simulink library "others"  (R2014a)
settings: Solver=ode45  StartTime=0.0  StopTime=10.0  RelTol=1e-3
undefined symbols (not defined in the file): n, num_closest_obstacles, TadjacencyMatrix, Tsim
settings Model: Creator=rspica  LastModifiedBy=rspica

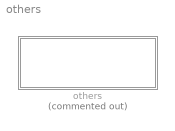
== system others ==
  others : Subsystem  Commented=on

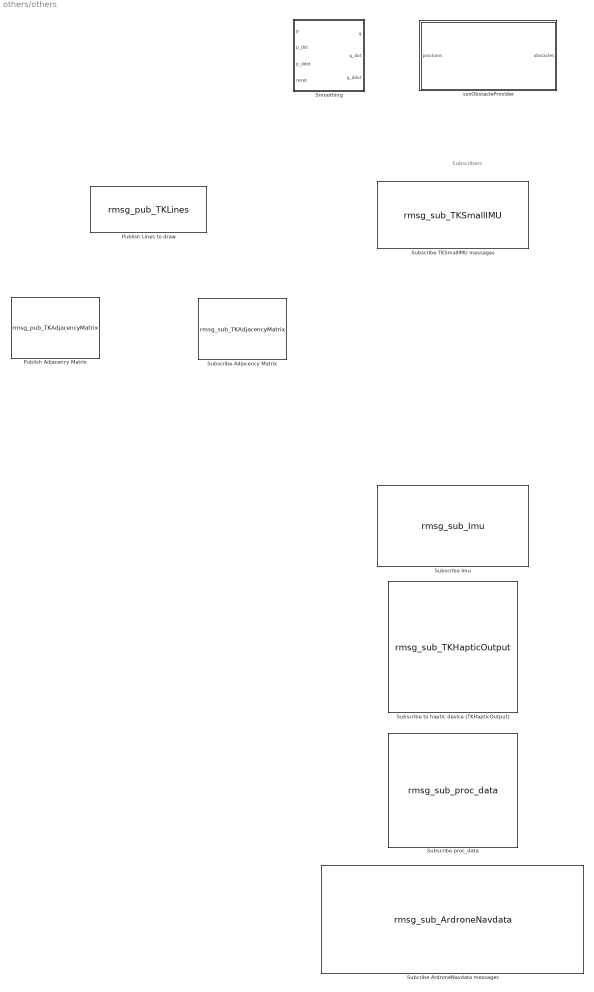
== system others/others ==
  note: Subscribers
  Publish Adjacency Matrix : S-Function  FunctionName=rmsg_pub_TKAdjacencyMatrix  Parameters=stepTime,topic  EnableBusSupport=off  mask{stepTime=TadjacencyMatrix, topic='/Matlab/AdjacencyMatrix'}
      mask prompts: stepTime "Simulation time step"; topic "ROS Topic"
      mask Display:
      | disp('Publish an\n\nAdjacency Matrix')
      | port_label('input', 1, 'A')
  Publish Lines to draw : S-Function  FunctionName=rmsg_pub_TKLines  Parameters=stepTime,topic  EnableBusSupport=off  mask(Line Drawer){stepTime=Tsim, topic='/TeleKyb/SwarmSimX/LineDrawer/input'}
      mask prompts: stepTime "Simulation time step"; topic "ROS Topic"
      mask help: This Block posts a collection of lines to the given ROS-Topic. Each line consists of a start- and destination-point in 3D and a color in 3D as RGB.
      mask Display:
      | disp('Line\nDrawer')
      | port_label('input', 1, 'start')
      | port_label('input', 2, 'destination')
      | port_label('input', 3, 'color')
  Smoothing : Subsystem  mask{time_to_95_percent=0.2}
      mask prompts: time_to_95_percent "Time in which 95% tracking should be reached"
      mask init:
      | A_smoothing = [0 0 0 0; 1 0 0 0; 0 1 0 0; 0 0 1 0];
      | B_smoothing = [1; 0; 0; 0];
      | dominant_pole = -3/time_to_95_percent;
      | p_smoothing = [dominant_pole, dominant_pole-1, dominant_pole-2, dominant_pole-3];
      | k_tracking = place(A_smoothing, B_smoothing, p_smoothing);
  "Subcribe ArdroneNavdata messages " : S-Function  FunctionName=rmsg_sub_ArdroneNavdata  Parameters=stepTime,topic_prefix,list_of_ids,topic_postfix  EnableBusSupport=off  mask{stepTime=Tsim, topic_prefix='/ardrone_', list_of_ids=uint32([0 1 2 3]), topic_postfix='/navdata'}
      mask prompts: stepTime "Simulation time step"; topic_prefix "ROS Topic (Prefix)"; list_of_ids "List of robot IDs (must be a vector of uint32)"; topic_postfix "ROS Topic (Postfix)"
      mask Display:
      | disp('Subscriber to \n ArdroneNavdata messages')
      | port_label('output',1,'magnetometer')
      | port_label('output',2,'pressure')
      | port_label('output',3,'temperature')
      | port_label('output',4,'rotation [degree angles]')
      | port_label('output',5,'altitude [cm]')
      | port_label('output',6,'velocity [mm/s]')
      | port_label('output',7,'raw vision velocity [mm/s]')
      | port_label('output',8,'accelerometers [g]')
      | port_label('output',9,'gyroscopes [deg/s]')
      | port_label('output',10,'vision state')
      | port_label('output',11,'state')
      | port_label('output',12,'battery level [%]')
      | port_label('output',13,'wind info')
      | port_label('output',14,'internal time')
      | port_label('output',15,'sent time')
  Subscribe Adjacency Matrix : S-Function  FunctionName=rmsg_sub_TKAdjacencyMatrix  Parameters=stepTime,topic,numRobots  EnableBusSupport=off  mask{stepTime=TadjacencyMatrix, topic='/Matlab/AdjacencyMatrix', numRobots=n}
      mask prompts: stepTime "Simulation time step"; topic "ROS Topic"; numRobots "number of robots"
      mask Display:
      | disp('Subscribe to\nAdjacency Matrix')
      | port_label('output', 1, 'A')
      | port_label('output', 2, 'sent time')
  Subscribe Imu : S-Function  FunctionName=rmsg_sub_Imu  Parameters=stepTime, topic_prefix,list_of_robot_ids,topic_postfix  EnableBusSupport=off  mask(Subscriber TKState){stepTime=Tsim, topic_prefix='/TeleKyb/SwarmSimX/Mikrokopter', list_of_robot_ids=uint32([0 1 2 3]), topic_postfix='/Sensor/VirtualIMU'}
      mask prompts: stepTime "Simulation time step"; topic_prefix "ROS Topic (Prefix)"; list_of_robot_ids "List of robot IDs (must be a uint32-Vector)"; topic_postfix "ROS Topic (Postfix)"
      mask help: ROS Subscriber Block for telekyb_msgs::TKState Messages
      mask Display:
      | disp('Subscribe to multiple\nTKImu messages')
      | port_label('output', 1, 'ang. vel.')
      | port_label('output', 2, 'lin. acc.')
      | port_label('output', 3, 'sent time')
  Subscribe TKSmallIMU messages : S-Function  FunctionName=rmsg_sub_TKSmallIMU  Parameters=stepTime,topic_prefix,list_of_ids,topic_postfix  EnableBusSupport=off  mask{stepTime=Tsim, topic_prefix='/TeleKyb/SmurfInterface_', list_of_ids=uint32([0 1 2 3]), topic_postfix='/Sensor/Imu'}
      mask prompts: stepTime "Simulation time step"; topic_prefix "ROS Topic (Prefix)"; list_of_ids "List of tobot IDs (must be a uint32-vector)"; topic_postfix "ROS Topic (Postfix)"
      mask Display:
      | disp('Subscriber to \n TKSmallIMU messages')
      | port_label('output',1,'ang. vel.')
      | port_label('output',2,'lin. acc.')
      | port_label('output',3,'sent time')
  Subscribe proc_data : S-Function  FunctionName=rmsg_sub_proc_data  Parameters=stepTime,topic_prefix,list_of_robot_ids,topic_postfix  EnableBusSupport=off  mask{stepTime=Tsim, topic_prefix='/TeleKyb/TeleKybCore_', list_of_robot_ids=uint32([0]), topic_postfix='/proc_data'}
      mask prompts: stepTime "Simulation time step"; topic_prefix "ROS Topic (Prefix)"; list_of_robot_ids "List of robot IDs (must be a uint32-Vector)"; topic_postfix "ROS Topic (Postfix)"
      mask Display:
      | disp('Subscribe to multiple\nproc_data messages')
      | port_label('output', 1, 'u')
      | port_label('output', 2, 'd')
      | port_label('output', 3, 'l')
      | port_label('output', 4, 'r')
      | port_label('output', 5, 'sent time')
  Subscribe to haptic device (TKHapticOutput) : S-Function  FunctionName=rmsg_sub_TKHapticOutput  Parameters=stepTime,topic  EnableBusSupport=off  mask{stepTime=Tsim, topic='/TeleKyb/Haptic/0/StatusOutput'}
      mask prompts: stepTime "Simulation time step"; topic "ROS Topic"
      mask Display:
      | disp('Subscriber to \n TKHapticOutput messages')
      | port_label('output',1,'position')
      | port_label('output',2,'orientation')
      | port_label('output',3,'linear velocity')
      | port_label('output',4,'force')
      | port_label('output',5,'loop frequency')
      | port_label('output',6,'primary button')
      | port_label('output',7,'sent time')
  ssxObstacleProvider : Subsystem  mask(SSX Obstacle Provider){stepTime=Tsim, topic_send='/TeleKyb/SwarmSimX/SegmentDistanceProvider/SegmentDefinition', topic_receive='/TeleKyb/SwarmSimX/SegmentDistanceProvider/SegmentDistanceProvider', num_robots=n, num_obstacles=num_closest_obstacles}
      mask prompts: stepTime "Simulation time step"; topic_send "ROS Topic to send to"; topic_receive "ROS Topic to receive from"; num_robots "Number of robots"; num_obstacles "Number of closest obstacles per segment that you want to receive"
      mask help:
      | You need to send the positions of the robots (a 3xn matrix) and get back the obstacles (in the form of a n x n x 7 x obs - matrix).
      | The 7 stands for:
      | 1: distance to obstacle
      | 2-4: closest point on the obstacle (x,y,z)
      | 5-7: closest point on the segment (x,y,z)
      |
      | So for example in the entry obstacles(1,2,3,4) there is:
      | the segment from robot 1 to robot 2 the y coordinate (see above) of the point on the closest obstacle with the number 4 (without any ordering of the obstacles, it's just one of the closest obstacles)
      mask Display:
      | disp('SSX Obstacle\n\n\nProvider')
      | port_label('input', 1, 'positions')
      | port_label('output', 1, 'obstacles')

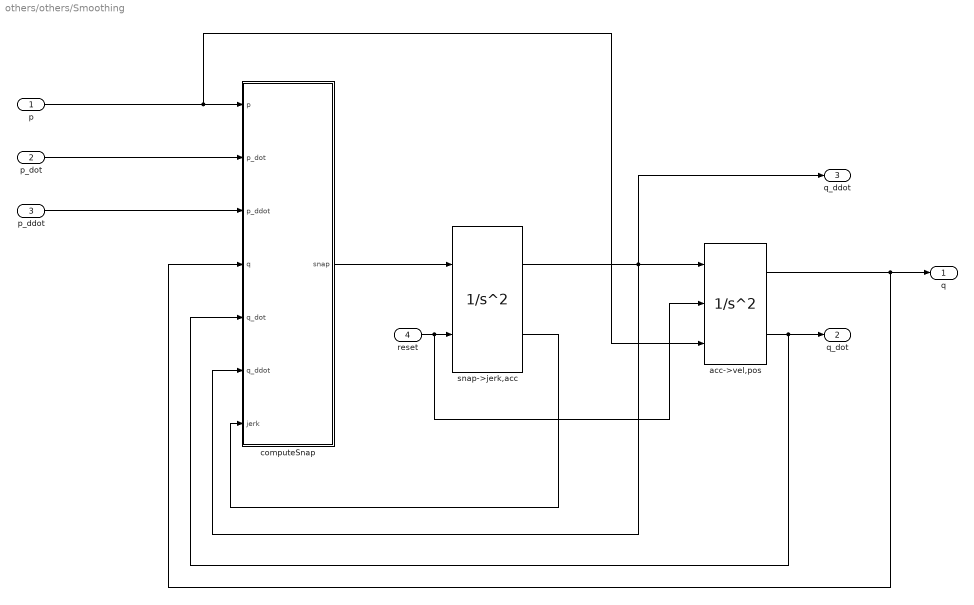
== system others/others/Smoothing ==
  p : Inport
  p_dot : Inport  Port=2
  p_ddot : Inport  Port=3
  reset : Inport  Port=4
  acc->vel,pos : SecondOrderIntegrator  ICSourceX=external  UpperLimitX=1  LowerLimitX=0  ICDXDT=0  ExternalReset=rising
  computeSnap : MATLAB Function  TreatAsAtomicUnit=on
  snap->jerk,acc : SecondOrderIntegrator  ICX=0  ICDXDT=0  ExternalReset=rising
  q : Outport
  q_dot : Outport  Port=2
  q_ddot : Outport  Port=3
  wires:
  acc->vel,pos/1 -> q/1, computeSnap/4(q)
  acc->vel,pos/2 -> q_dot/1, computeSnap/5(q_dot)
  p_dot/1 -> computeSnap/2(p_dot)
  snap->jerk,acc/1 -> acc->vel,pos/1, q_ddot/1, computeSnap/6(q_ddot)
  reset/1 -> acc->vel,pos/2, snap->jerk,acc/2
  p/1 -> computeSnap/1(p), acc->vel,pos/3
  p_ddot/1 -> computeSnap/3(p_ddot)
  snap->jerk,acc/2 -> computeSnap/7(jerk)
  computeSnap/1(snap) -> snap->jerk,acc/1

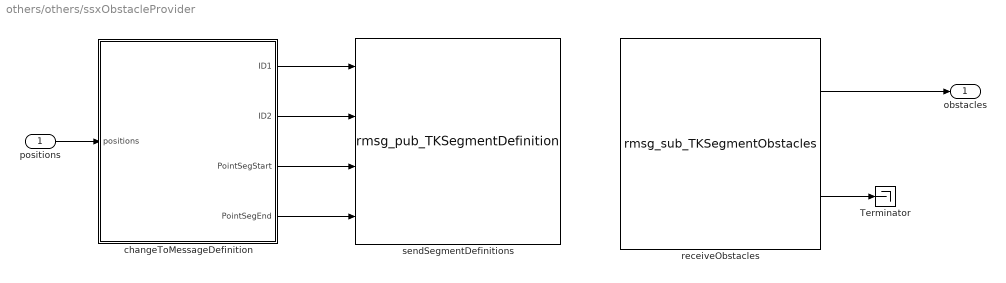
== system others/others/ssxObstacleProvider ==
  positions : Inport
  Terminator : Terminator
  changeToMessageDefinition : MATLAB Function  TreatAsAtomicUnit=on
  receiveObstacles : S-Function  FunctionName=rmsg_sub_TKSegmentObstacles  Parameters=stepTime,topic_receive,num_robots,num_obstacles  EnableBusSupport=off
  sendSegmentDefinitions : S-Function  FunctionName=rmsg_pub_TKSegmentDefinition  Parameters=stepTime,topic_send  EnableBusSupport=off
  obstacles : Outport
  wires:
  changeToMessageDefinition/4(PointSegEnd) -> sendSegmentDefinitions/4
  changeToMessageDefinition/3(PointSegStart) -> sendSegmentDefinitions/3
  changeToMessageDefinition/2(ID2) -> sendSegmentDefinitions/2
  changeToMessageDefinition/1(ID1) -> sendSegmentDefinitions/1
  receiveObstacles/2 -> Terminator/1
  receiveObstacles/1 -> obstacles/1
  positions/1 -> changeToMessageDefinition/1(positions)

== matlab function others/Smoothing/computeSnap ==
  data: p input; p_dot input; p_ddot input; q input; q_dot input; q_ddot input; jerk input; k_tracking parameter size=4; snap output
function snap = fcn(p,p_dot,p_ddot,q,q_dot,q_ddot,jerk,k_tracking)
%#codegen

snap = k_tracking(1) * (-jerk) + k_tracking(2) * (p_ddot - q_ddot) + k_tracking(3) * (p_dot - q_dot) + k_tracking(4) * (p - q);


end

== matlab function others/ssxObstacleProvider/changeToMessageDefinition ==
  settings: updateMethod=DISCRETE  sampleTime=stepTime
  data: positions input; n parameter; ID1 output; ID2 output; PointSegStart output; PointSegEnd output
function [ID1, ID2, PointSegStart, PointSegEnd] = getClosestObstacles(positions,n)
% Obstacle Provider

num_segments = n*(n-1)/2;
dID1 = zeros(num_segments,1);
dID2 = zeros(num_segments,1);
PointSegStart = zeros(3,num_segments);
PointSegEnd = zeros(3,num_segments);

counter = 1;
for i = 1:n
    for j= i+1:n
        dID1(counter) = i;
        dID2(counter) = j;
        PointSegStart(:,counter) = positions(:,i);
        PointSegEnd(:,counter) = positions(:,j);
        counter = counter + 1;
    end
end

ID1 = uint8(dID1);
ID2 = uint8(dID2);
